simulink model "MPC"  (R2024b)
settings: Solver=ode4  StartTime=0.0  StopTime=tsim  FixedStep=baseRate  RelTol=1e-6  AbsTol=1e-6
values from neighbouring files (symbols this model uses):
  IBLACK = 0.1996    [unpackData.m]
  IRED = 0.1982    [unpackData.m]
  m = m + 5    (= 4)    [unpackData.m]
  M = diag([1/m; 1/m; 1/I])    [unpackData.m]
  mBLACK = 11.3620    (= 11.362)    [unpackData.m]
  mRED = 11.2970    (= 11.297)    [unpackData.m]
  N = 0    [unpackData.m]
  Q = blkdiag(0.0001*eye(2), 0.00001)    [unpackData.m]
  R = diag([6;6;6])    [unpackData.m]
undefined symbols (not defined in the file or in its folder): a1, a2, a3, alpha, alpha_m, alpha_t, alphas, alphas_t, alphat, Am, b, b0, b1, b2, b3, baseRate, Bm, C, c, c1, c1t, c2, c2t, camera_FOV, camera_offset, Cm, d, dataRate, DiscIntNeverNeededParam, Dm, docking_face, docking_offset, drop_states_ARM, drop_states_BLACK, drop_states_BLUE, drop_states_RED, epsilon, epsilont, eta, F_black_X_nominal, F_black_Y_nominal, F_blue_X_nominal, F_blue_Y_nominal, F_max, F_red_X_nominal, F_red_Y_nominal, f_t, F_t, F_thrusters_BLACK, F_thrusters_BLUE, F_thrusters_RED, F_u, f_u, F_v, gamma, Gamma1_el, Gamma1_sh, Gamma1_wr, Gamma2_el, Gamma2_sh ... (+118)
libraries: simulink x33, nvidiaSharedBlocks x13, slpidlib x6, MainLibrary x5, dspsigops x3, dspinverses x3, nvidiaIMUSensorslib x1
(part 6 of 11)

== system MPC/4 - Control/Default PD Control (RED)/Calculate Error ==
  Desired Attitude : Inport
  Measured Attitude : Inport  Port=2
  MATLAB Function : MATLAB Function  TreatAsAtomicUnit=on
  Attitude Error : Outport
  wires:
  MATLAB Function/1(Rz_error) -> Attitude Error/1
  Desired Attitude/1 -> MATLAB Function/1(Rz_path)
  Measured Attitude/1 -> MATLAB Function/2(Rz_measured)

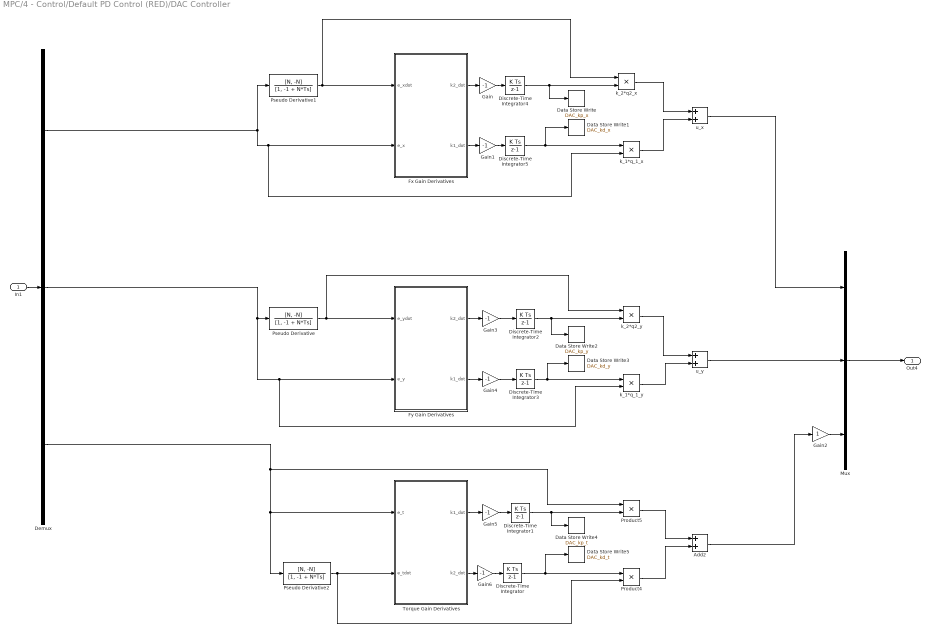
== system MPC/4 - Control/Default PD Control (RED)/DAC Controller ==
  In1 : Inport
  Add2 : Sum
  Data Store Write : DataStoreWrite  DataStoreName=DAC_kp_x  IndexOptions=Index vector (dialog)  Indices=1  OutputSizes=1
  Data Store Write1 : DataStoreWrite  DataStoreName=DAC_kd_x  IndexOptions=Index vector (dialog)  Indices=1  OutputSizes=1
  Data Store Write2 : DataStoreWrite  DataStoreName=DAC_kp_y  IndexOptions=Index vector (dialog)  Indices=1  OutputSizes=1
  Data Store Write3 : DataStoreWrite  DataStoreName=DAC_kd_y  IndexOptions=Index vector (dialog)  Indices=1  OutputSizes=1
  Data Store Write4 : DataStoreWrite  DataStoreName=DAC_kp_t  IndexOptions=Index vector (dialog)  Indices=1  OutputSizes=1
  Data Store Write5 : DataStoreWrite  DataStoreName=DAC_kd_t  IndexOptions=Index vector (dialog)  Indices=1  OutputSizes=1
  Demux : Demux  Outputs=3
  Discrete-Time Integrator : DiscreteIntegrator  InitialCondition=k_2_t_0  SampleTime=-1  ICPrevOutput=DiscIntNeverNeededParam  ICPrevScaledInput=DiscIntNeverNeededParam
  Discrete-Time Integrator1 : DiscreteIntegrator  InitialCondition=k_1_t_0  SampleTime=-1  ICPrevOutput=DiscIntNeverNeededParam  ICPrevScaledInput=DiscIntNeverNeededParam
  Discrete-Time Integrator2 : DiscreteIntegrator  InitialCondition=k_2_0  SampleTime=-1  ICPrevOutput=DiscIntNeverNeededParam  ICPrevScaledInput=DiscIntNeverNeededParam
  Discrete-Time Integrator3 : DiscreteIntegrator  InitialCondition=k_1_0  SampleTime=-1  ICPrevOutput=DiscIntNeverNeededParam  ICPrevScaledInput=DiscIntNeverNeededParam
  Discrete-Time Integrator4 : DiscreteIntegrator  InitialCondition=k_2_0  SampleTime=-1  ICPrevOutput=DiscIntNeverNeededParam  ICPrevScaledInput=DiscIntNeverNeededParam
  Discrete-Time Integrator5 : DiscreteIntegrator  InitialCondition=k_1_0  SampleTime=-1  ICPrevOutput=DiscIntNeverNeededParam  ICPrevScaledInput=DiscIntNeverNeededParam
  Fx Gain Derivatives : MATLAB Function  TreatAsAtomicUnit=on
  Fy Gain Derivatives : MATLAB Function  TreatAsAtomicUnit=on
  Gain{,1,3..6} (6 alike) : Gain  Gain=-1
  Gain2 : Gain
  Mux : Mux  Inputs=3
  Product4 : Product
  Product5 : Product
  Pseudo Derivative : DiscreteTransferFcn  Numerator=[N, -N]  Denominator=[1, -1 + N*Ts]
  Pseudo Derivative1 : DiscreteTransferFcn  Numerator=[N, -N]  Denominator=[1, -1 + N*Ts]
  Pseudo Derivative2 : DiscreteTransferFcn  Numerator=[N, -N]  Denominator=[1, -1 + N*Ts]
  Torque Gain Derivatives : MATLAB Function  TreatAsAtomicUnit=on
  k_1*q_1_x : Product
  k_1*q_1_y : Product
  k_2*q2_x : Product
  k_2*q2_y : Product
  u_x : Sum
  u_y : Sum
  Out4 : Outport
  wires:
  Add2/1 -> Gain2/1
  u_y/1 -> Mux/2
  Pseudo Derivative/1 -> k_2*q2_y/1, Fy Gain Derivatives/1(e_ydot)
  Demux/2 -> Fy Gain Derivatives/2(e_y), k_1*q_1_y/2, Pseudo Derivative/1
  k_2*q2_y/1 -> u_y/1
  Fy Gain Derivatives/2(k1_dot) -> Gain4/1
  k_1*q_1_y/1 -> u_y/2
  Fy Gain Derivatives/1(k2_dot) -> Gain3/1
  Torque Gain Derivatives/1(k1_dot) -> Gain5/1
  Pseudo Derivative2/1 -> Torque Gain Derivatives/2(e_tdot), Product4/2
  Product5/1 -> Add2/1
  Product4/1 -> Add2/2
  Torque Gain Derivatives/2(k2_dot) -> Gain6/1
  Demux/1 -> k_1*q_1_x/2, Fx Gain Derivatives/2(e_x), Pseudo Derivative1/1
  Pseudo Derivative1/1 -> k_2*q2_x/1, Fx Gain Derivatives/1(e_xdot)
  k_1*q_1_x/1 -> u_x/2
  u_x/1 -> Mux/1
  k_2*q2_x/1 -> u_x/1
  Demux/3 -> Torque Gain Derivatives/1(e_t), Pseudo Derivative2/1, Product5/1
  In1/1 -> Demux/1
  Mux/1 -> Out4/1
  Gain2/1 -> Mux/3
  Discrete-Time Integrator2/1 -> Data Store Write2/1, k_2*q2_y/2
  Discrete-Time Integrator5/1 -> Data Store Write1/1, k_1*q_1_x/1
  Discrete-Time Integrator4/1 -> Data Store Write/1, k_2*q2_x/2
  Discrete-Time Integrator1/1 -> Data Store Write4/1, Product5/2
  Fx Gain Derivatives/1(k2_dot) -> Gain/1
  Fx Gain Derivatives/2(k1_dot) -> Gain1/1
  Gain/1 -> Discrete-Time Integrator4/1
  Gain1/1 -> Discrete-Time Integrator5/1
  Gain3/1 -> Discrete-Time Integrator2/1
  Gain4/1 -> Discrete-Time Integrator3/1
  Gain5/1 -> Discrete-Time Integrator1/1
  Gain6/1 -> Discrete-Time Integrator/1
  Discrete-Time Integrator3/1 -> Data Store Write3/1, k_1*q_1_y/1
  Discrete-Time Integrator/1 -> Data Store Write5/1, Product4/1

== system MPC/4 - Control/Default PD Control (RED)/Diff ==
  In1 : Inport
  In2 : Inport  Port=2
  Demux : Demux  Outputs=3
  Demux1 : Demux  Outputs=3
  Hough Control : Subsystem
      settings: PortSchema="{\"entries\":[{\"content\":{\"sides\":[{\"content\":{\"connectorIds\":[\"In1\"]},\"type\":\"ConnectorPlacement.EquallySpacedRectSide\",\"uuid\":\"a8dcddb7-9836-4673-8356-a3c89c9502b3\"},{\"content\":{\"connectorIds\":[\"Out1\"],\"side\":\"RIGHT\"},\"type\":\"ConnectorPlacement.EquallySpacedRectSide\",\"uuid\":\"2c97d3bb-11f9-4ba2-b448-09694ac8e6f8\"},{\"content\":{\"side\":\"TOP\"},\"type\":\"ConnectorPlacement.EquallySpacedRectSide\",\"uuid\":\"bc41882c-3443-497d-b6f8-69c8cbf4c339\"},{\"content\":{\"connectorIds\":[\"In2\"],\"side\":\"BOTTOM\"},\"type\":\"ConnectorPlacement.EquallySpacedRectSide\",\"uuid\":\"14b1077a-07d2-46a7-87f1-61ebe292854a\"}]},\"type\":\"ConnectorPlacement.EquallySpacedConnector\",\"uuid\":\"2f9ed5e7-457a-4e66-9582-5133e2ff8cc8\"}],\"packageUris\":[\"http://schema.mathworks.com/mf0/Connector/R2020b\"],\"version\":\"1.0\"}"
  Mux : Mux  Inputs=3
  Sum : Sum  Inputs=|+-
  Sum1 : Sum  Inputs=|+-
  u : Outport
  wires:
  In1/1 -> Demux/1
  Demux/2 -> Sum/1
  Demux/1 -> Sum1/1
  In2/1 -> Demux1/1
  Demux1/1 -> Sum1/2
  Demux1/2 -> Sum/2
  Demux/3 -> Hough Control/1(Ref)
  Demux1/3 -> Hough Control/2(Act)
  Hough Control/1(Err) -> Mux/3
  Sum/1 -> Mux/2
  Sum1/1 -> Mux/1
  Mux/1 -> u/1

== system MPC/4 - Control/Default PD Control (RED)/H_inf ==
  In1 : Inport
  Demux : Demux  Outputs=3
  Discrete State-Space : DiscreteStateSpace  A=K.A  B=K.B  C=K.C  D=K.D  SampleTime=-1
  Discrete State-Space1 : DiscreteStateSpace  A=K_t.A  B=K_t.B  C=K_t.C  D=K_t.D  SampleTime=-1
  Discrete State-Space2 : DiscreteStateSpace  A=K.A  B=K.B  C=K.C  D=K.D  SampleTime=-1
  Mux : Mux  Inputs=3
  Out1 : Outport
  wires:
  In1/1 -> Demux/1
  Mux/1 -> Out1/1
  Demux/3 -> Discrete State-Space1/1
  Discrete State-Space1/1 -> Mux/3
  Demux/1 -> Discrete State-Space/1
  Discrete State-Space/1 -> Mux/1
  Demux/2 -> Discrete State-Space2/1
  Discrete State-Space2/1 -> Mux/2

== system MPC/4 - Control/Default PD Control (RED)/Homo ==
  In1 : Inport
  Demux : Demux  Outputs=3
  MATLAB Function : MATLAB Function  TreatAsAtomicUnit=on
  MATLAB Function1 : MATLAB Function  TreatAsAtomicUnit=on
  MATLAB Function2 : MATLAB Function  TreatAsAtomicUnit=on
  MATLAB Function3 : MATLAB Function  TreatAsAtomicUnit=on
  MATLAB Function4 : MATLAB Function  TreatAsAtomicUnit=on
  MATLAB Function5 : MATLAB Function  TreatAsAtomicUnit=on
  Mux : Mux  Inputs=3
  Pseudo Derivative : DiscreteTransferFcn  Numerator=[N, -N]  Denominator=[1, -1 + N*Ts]
  Pseudo Derivative1 : DiscreteTransferFcn  Numerator=[N, -N]  Denominator=[1, -1 + N*Ts]
  Pseudo Derivative2 : DiscreteTransferFcn  Numerator=[N, -N]  Denominator=[1, -1 + N*Ts]
  Sum : Sum  Inputs=++|
  Sum1 : Sum  Inputs=++|
  Sum2 : Sum  Inputs=++|
  Out1 : Outport
  wires:
  Demux/1 -> Pseudo Derivative/1, MATLAB Function/1(q1)
  Pseudo Derivative/1 -> MATLAB Function1/1(q2)
  Sum/1 -> Mux/1
  MATLAB Function/1(u) -> Sum/1
  MATLAB Function1/1(u) -> Sum/2
  Pseudo Derivative1/1 -> MATLAB Function3/1(q2)
  Sum1/1 -> Mux/2
  MATLAB Function3/1(u) -> Sum1/2
  Demux/2 -> MATLAB Function2/1(q1), Pseudo Derivative1/1
  MATLAB Function2/1(u) -> Sum1/1
  Demux/3 -> MATLAB Function4/1(q1), Pseudo Derivative2/1
  Pseudo Derivative2/1 -> MATLAB Function5/1(q2)
  MATLAB Function5/1(u) -> Sum2/2
  MATLAB Function4/1(u) -> Sum2/1
  Sum2/1 -> Mux/3
  Mux/1 -> Out1/1
  In1/1 -> Demux/1

== system MPC/4 - Control/Default PD Control (RED)/LQR ==
  In1 : Inport
  Constant : Constant  Value=k
  Demux : Demux  Outputs=3
  MATLAB Function : MATLAB Function  TreatAsAtomicUnit=on
  Pseudo Derivative : DiscreteTransferFcn  Numerator=[N, -N]  Denominator=[1, -1 + N*Ts]
  Pseudo Derivative1 : DiscreteTransferFcn  Numerator=[N, -N]  Denominator=[1, -1 + N*Ts]
  Pseudo Derivative2 : DiscreteTransferFcn  Numerator=[N, -N]  Denominator=[1, -1 + N*Ts]
  Out1 : Outport
  wires:
  Constant/1 -> MATLAB Function/1(k)
  MATLAB Function/1(u) -> Out1/1
  Demux/3 -> Pseudo Derivative2/1, MATLAB Function/6(q1_t)
  Demux/2 -> Pseudo Derivative1/1, MATLAB Function/4(q1_y)
  Demux/1 -> Pseudo Derivative/1, MATLAB Function/2(q1_x)
  Pseudo Derivative2/1 -> MATLAB Function/7(q2_t)
  Pseudo Derivative/1 -> MATLAB Function/3(q2_x)
  Pseudo Derivative1/1 -> MATLAB Function/5(q2_y)
  In1/1 -> Demux/1

== system MPC/4 - Control/Default PD Control (RED)/Min Energy ==
  In1 : Inport
  Clock : Clock
  Clock1 : Clock
  Clock2 : Clock
  Demux : Demux  Outputs=3
  MATLAB Function : MATLAB Function  TreatAsAtomicUnit=on
  MATLAB Function1 : MATLAB Function  TreatAsAtomicUnit=on
  MATLAB Function2 : MATLAB Function  TreatAsAtomicUnit=on
  Mux : Mux  Inputs=3
  Pseudo Derivative : DiscreteTransferFcn  Numerator=[N, -N]  Denominator=[1, -1 + N*Ts]
  Pseudo Derivative1 : DiscreteTransferFcn  Numerator=[N, -N]  Denominator=[1, -1 + N*Ts]
  Pseudo Derivative2 : DiscreteTransferFcn  Numerator=[N, -N]  Denominator=[1, -1 + N*Ts]
  Subsystem : Subsystem
  Subsystem1 : Subsystem
  Subsystem2 : Subsystem
  Sum : Sum  Inputs=|++
  Sum1 : Sum  Inputs=|++
  Sum2 : Sum  Inputs=|++
  Out1 : Outport
  wires:
  Demux/2 -> Subsystem1/2(u), Pseudo Derivative1/1, MATLAB Function/1(q1)
  Pseudo Derivative1/1 -> MATLAB Function/2(q2)
  Clock/1 -> MATLAB Function/3(t)
  MATLAB Function/1(u) -> Sum1/1
  Clock1/1 -> MATLAB Function1/3(t)
  Pseudo Derivative/1 -> MATLAB Function1/2(q2)
  MATLAB Function1/1(u) -> Sum/1
  Demux/1 -> Subsystem/2(u), MATLAB Function1/1(q1), Pseudo Derivative/1
  Clock2/1 -> MATLAB Function2/3(t)
  Pseudo Derivative2/1 -> MATLAB Function2/2(q2)
  MATLAB Function2/1(u) -> Sum2/1
  Demux/3 -> Subsystem2/2(u), Pseudo Derivative2/1, MATLAB Function2/1(q1)
  Mux/1 -> Out1/1
  In1/1 -> Demux/1
  MATLAB Function1/2(dt) -> Subsystem/1(In2)
  Sum/1 -> Mux/1
  Subsystem/1(Out1) -> Sum/2
  MATLAB Function/2(dt) -> Subsystem1/1(dt)
  Sum1/1 -> Mux/2
  Subsystem1/1(Out1) -> Sum1/2
  Sum2/1 -> Mux/3
  Subsystem2/1(Out1) -> Sum2/2
  MATLAB Function2/2(dt) -> Subsystem2/1(dt)

== system MPC/4 - Control/Default PD Control (RED)/Minimum Time Controller ==
  In1 : Inport
  Demux : Demux  Outputs=3
  Gain : Gain  Gain=F_max
  Gain1 : Gain  Gain=F_max
  Gain2 : Gain  Gain=T_max
  MATLAB Function : MATLAB Function  TreatAsAtomicUnit=on
  MATLAB Function1 : MATLAB Function  TreatAsAtomicUnit=on
  MATLAB Function2 : MATLAB Function  TreatAsAtomicUnit=on
  MATLAB Function3 : MATLAB Function  TreatAsAtomicUnit=on
  MATLAB Function4 : MATLAB Function  TreatAsAtomicUnit=on
  MATLAB Function5 : MATLAB Function  TreatAsAtomicUnit=on
  Mux : Mux  Inputs=3
  Pseudo Derivative : DiscreteTransferFcn  Numerator=[N, -N]  Denominator=[1, -1 + N*Ts]
  Pseudo Derivative1 : DiscreteTransferFcn  Numerator=[N, -N]  Denominator=[1, -1 + N*Ts]
  Pseudo Derivative2 : DiscreteTransferFcn  Numerator=[N, -N]  Denominator=[1, -1 + N*Ts]
  Out1 : Outport
  wires:
  Demux/1 -> MATLAB Function/1(q_1), MATLAB Function3/1(q_1), Pseudo Derivative/1
  Demux/3 -> Pseudo Derivative2/1, MATLAB Function2/1(q_1), MATLAB Function5/1(q_1)
  Pseudo Derivative/1 -> MATLAB Function/2(q_2)
  Demux/2 -> Pseudo Derivative1/1, MATLAB Function4/1(q_1), MATLAB Function1/1(q_1)
  Pseudo Derivative1/1 -> MATLAB Function1/2(q_2)
  Pseudo Derivative2/1 -> MATLAB Function2/2(q_2)
  MATLAB Function/1(sign_Argument) -> MATLAB Function3/2(sign_Argument)
  MATLAB Function1/1(sign_Argument) -> MATLAB Function4/2(sign_Argument)
  MATLAB Function2/1(sign_Argument) -> MATLAB Function5/2(sign_Argument)
  MATLAB Function3/1(u_max_product) -> Gain/1
  Gain/1 -> Mux/1
  MATLAB Function4/1(u_max_product) -> Gain1/1
  Gain1/1 -> Mux/2
  MATLAB Function5/1(u_max_product) -> Gain2/1
  Gain2/1 -> Mux/3
  In1/1 -> Demux/1
  Mux/1 -> Out1/1

== system MPC/4 - Control/Default PD Control (RED)/PD ==
  In1 : Inport
  Demux : Demux  Outputs=3
  Mux : Mux  Inputs=3
  PID Controller1 : slpidlib/PID Controller  Controller=PD  Form=Parallel  TimeDomain=Discrete-time  UseExternalTs=off  SampleTime=-1  IntegratorMethod=Forward Euler  FilterMethod=Forward Euler  ControllerParametersSource=internal  P=k_p  I=1  UseKiTs=off  D=k_d  N=N  UseFilter=on  TunerSelectOption=Transfer Function Based (PID Tuner App)  InitialConditionSource=internal  InitialConditionForIntegrator=0  InitialConditionForFilter=0  DifferentiatorICPrevScaledInput=0  ExternalReset=none  TrackingMode=off  Kt=1  LimitOutput=off  SatLimitsSource=internal  UpperSaturationLimit=inf  LowerSaturationLimit=-inf  LinearizeAsGain=on  AntiWindupMode=none  Kb=1  LimitIntegrator=off  UpperIntegratorSaturationLimit=inf  LowerIntegratorSaturationLimit=-inf  POutMin=[]  POutMax=[]  IOutMin=[]  IOutMax=[]  DOutMin=[]  DOutMax=[]  NOutMin=[]  NOutMax=[]  SumOutMin=[]  SumOutMax=[]  SaturationOutMin=[]  SaturationOutMax=[]  PParamMin=[]  PParamMax=[]  IParamMin=[]  IParamMax=[]  DParamMin=[]  DParamMax=[]  NParamMin=[]  NParamMax=[]  KbParamMin=[]  KbParamMax=[]  KtParamMin=[]  KtParamMax=[]  KbOutMin=[]  KbOutMax=[]  KtOutMin=[]  KtOutMax=[]  IntegratorOutMin=[]  IntegratorOutMax=[]  FilterOutMin=[]  FilterOutMax=[]  SumI1OutMin=[]  SumI1OutMax=[]  SumI2OutMin=[]  SumI2OutMax=[]  SumI3OutMin=[]  SumI3OutMax=[]  SumI4OutMin=[]  SumI4OutMax=[]  SumDOutMin=[]  SumDOutMax=[]  DifferentiatorOutMin=[]  DifferentiatorOutMax=[]  FilterDiffOutCoefMin=[]  FilterDiffOutCoefMax=[]  ReciprocalOutMin=[]  ReciprocalOutMax=[]  SumDenOutMin=[]  SumDenOutMax=[]  SumNumOutMin=[]  SumNumOutMax=[]  DivideOutMin=[]  DivideOutMax=[]  UdiffTsProdOutMin=[]  UdiffTsProdOutMax=[]  NTsProdOutMin=[]  NTsProdOutMax=[]  UintegralTsProdOutMin=[]  UintegralTsProdOutMax=[]  UngainTsProdOutMin=[]  UngainTsProdOutMax=[]  ClampingZeroOutDataTypeStr=Inherit: Inherit via back propagation  ClampingZeroOutMin=[]  ClampingZeroOutMax=[]  FilterDenConstantOutDataTypeStr=Inherit: Inherit via back propagation  FilterDenConstantOutMin=[]  FilterDenConstantOutMax=[]  PCopyOutDataTypeStr=Inherit: Inherit via back propagation  PCopyOutMin=[]  PCopyOutMax=[]  NCopyOutDataTypeStr=Inherit: Inherit via back propagation  NCopyOutMin=[]  NCopyOutMax=[]  IntegratorContinuousStateAttributes=''  IntegratorStateMustResolveToSignalObject=off  IntegratorRTWStateStorageClass=Auto  FilterContinuousStateAttributes=''  FilterStateMustResolveToSignalObject=off  FilterRTWStateStorageClass=Auto  ParallelPVariant=InternalParameters  IdealPVariant=Disabled  IVariant=Disabled  DVariant=InternalParameters  IntegratorVariant=Disabled  SatVariant=Disabled  AWVariant=Disabled  PCopyVariant=Disabled  TRVariant=Disabled  FdbkBlocksVariant=Forward  IdealPFdbkVariant=Disabled  SatFdbkVariant=Disabled  DerivativeFilterVariant=ForwardEulerFilter  NVariant=InternalParameters  NCopyVariant=Disabled  FilterICVariant=InternalICsFilter  IntegratorICVariant=Disabled  ExternalResetVariant=Disabled  TRSumVariant=Passthrough  SumFdbkVariant=Disabled  SumVariant=Sum_PD  TsampFilterVariant=InternalTs  TsampNgainVariant=Passthrough  TsampIntegralVariant=Disabled_SignalSpec  ExternalSaturationOutDataTypeStr=Inherit: Same as second input
  PID Controller2 : slpidlib/PID Controller  Controller=PD  Form=Parallel  TimeDomain=Discrete-time  UseExternalTs=off  SampleTime=-1  IntegratorMethod=Forward Euler  FilterMethod=Forward Euler  ControllerParametersSource=internal  P=k_p  I=1  UseKiTs=off  D=k_d  N=N  UseFilter=on  TunerSelectOption=Transfer Function Based (PID Tuner App)  InitialConditionSource=internal  InitialConditionForIntegrator=0  InitialConditionForFilter=0  DifferentiatorICPrevScaledInput=0  ExternalReset=none  TrackingMode=off  Kt=1  LimitOutput=off  SatLimitsSource=internal  UpperSaturationLimit=inf  LowerSaturationLimit=-inf  LinearizeAsGain=on  AntiWindupMode=none  Kb=1  LimitIntegrator=off  UpperIntegratorSaturationLimit=inf  LowerIntegratorSaturationLimit=-inf  POutMin=[]  POutMax=[]  IOutMin=[]  IOutMax=[]  DOutMin=[]  DOutMax=[]  NOutMin=[]  NOutMax=[]  SumOutMin=[]  SumOutMax=[]  SaturationOutMin=[]  SaturationOutMax=[]  PParamMin=[]  PParamMax=[]  IParamMin=[]  IParamMax=[]  DParamMin=[]  DParamMax=[]  NParamMin=[]  NParamMax=[]  KbParamMin=[]  KbParamMax=[]  KtParamMin=[]  KtParamMax=[]  KbOutMin=[]  KbOutMax=[]  KtOutMin=[]  KtOutMax=[]  IntegratorOutMin=[]  IntegratorOutMax=[]  FilterOutMin=[]  FilterOutMax=[]  SumI1OutMin=[]  SumI1OutMax=[]  SumI2OutMin=[]  SumI2OutMax=[]  SumI3OutMin=[]  SumI3OutMax=[]  SumI4OutMin=[]  SumI4OutMax=[]  SumDOutMin=[]  SumDOutMax=[]  DifferentiatorOutMin=[]  DifferentiatorOutMax=[]  FilterDiffOutCoefMin=[]  FilterDiffOutCoefMax=[]  ReciprocalOutMin=[]  ReciprocalOutMax=[]  SumDenOutMin=[]  SumDenOutMax=[]  SumNumOutMin=[]  SumNumOutMax=[]  DivideOutMin=[]  DivideOutMax=[]  UdiffTsProdOutMin=[]  UdiffTsProdOutMax=[]  NTsProdOutMin=[]  NTsProdOutMax=[]  UintegralTsProdOutMin=[]  UintegralTsProdOutMax=[]  UngainTsProdOutMin=[]  UngainTsProdOutMax=[]  ClampingZeroOutDataTypeStr=Inherit: Inherit via back propagation  ClampingZeroOutMin=[]  ClampingZeroOutMax=[]  FilterDenConstantOutDataTypeStr=Inherit: Inherit via back propagation  FilterDenConstantOutMin=[]  FilterDenConstantOutMax=[]  PCopyOutDataTypeStr=Inherit: Inherit via back propagation  PCopyOutMin=[]  PCopyOutMax=[]  NCopyOutDataTypeStr=Inherit: Inherit via back propagation  NCopyOutMin=[]  NCopyOutMax=[]  IntegratorContinuousStateAttributes=''  IntegratorStateMustResolveToSignalObject=off  IntegratorRTWStateStorageClass=Auto  FilterContinuousStateAttributes=''  FilterStateMustResolveToSignalObject=off  FilterRTWStateStorageClass=Auto  ParallelPVariant=InternalParameters  IdealPVariant=Disabled  IVariant=Disabled  DVariant=InternalParameters  IntegratorVariant=Disabled  SatVariant=Disabled  AWVariant=Disabled  PCopyVariant=Disabled  TRVariant=Disabled  FdbkBlocksVariant=Forward  IdealPFdbkVariant=Disabled  SatFdbkVariant=Disabled  DerivativeFilterVariant=ForwardEulerFilter  NVariant=InternalParameters  NCopyVariant=Disabled  FilterICVariant=InternalICsFilter  IntegratorICVariant=Disabled  ExternalResetVariant=Disabled  TRSumVariant=Passthrough  SumFdbkVariant=Disabled  SumVariant=Sum_PD  TsampFilterVariant=InternalTs  TsampNgainVariant=Passthrough  TsampIntegralVariant=Disabled_SignalSpec  ExternalSaturationOutDataTypeStr=Inherit: Same as second input
  PID Controller3 : slpidlib/PID Controller  Controller=PD  Form=Parallel  TimeDomain=Discrete-time  UseExternalTs=off  SampleTime=-1  IntegratorMethod=Forward Euler  FilterMethod=Forward Euler  ControllerParametersSource=internal  P=k_p_t  I=1  UseKiTs=off  D=k_d_t  N=100  UseFilter=on  TunerSelectOption=Transfer Function Based (PID Tuner App)  InitialConditionSource=internal  InitialConditionForIntegrator=0  InitialConditionForFilter=0  DifferentiatorICPrevScaledInput=0  ExternalReset=none  TrackingMode=off  Kt=1  LimitOutput=off  SatLimitsSource=internal  UpperSaturationLimit=inf  LowerSaturationLimit=-inf  LinearizeAsGain=on  AntiWindupMode=none  Kb=1  LimitIntegrator=off  UpperIntegratorSaturationLimit=inf  LowerIntegratorSaturationLimit=-inf  POutMin=[]  POutMax=[]  IOutMin=[]  IOutMax=[]  DOutMin=[]  DOutMax=[]  NOutMin=[]  NOutMax=[]  SumOutMin=[]  SumOutMax=[]  SaturationOutMin=[]  SaturationOutMax=[]  PParamMin=[]  PParamMax=[]  IParamMin=[]  IParamMax=[]  DParamMin=[]  DParamMax=[]  NParamMin=[]  NParamMax=[]  KbParamMin=[]  KbParamMax=[]  KtParamMin=[]  KtParamMax=[]  KbOutMin=[]  KbOutMax=[]  KtOutMin=[]  KtOutMax=[]  IntegratorOutMin=[]  IntegratorOutMax=[]  FilterOutMin=[]  FilterOutMax=[]  SumI1OutMin=[]  SumI1OutMax=[]  SumI2OutMin=[]  SumI2OutMax=[]  SumI3OutMin=[]  SumI3OutMax=[]  SumI4OutMin=[]  SumI4OutMax=[]  SumDOutMin=[]  SumDOutMax=[]  DifferentiatorOutMin=[]  DifferentiatorOutMax=[]  FilterDiffOutCoefMin=[]  FilterDiffOutCoefMax=[]  ReciprocalOutMin=[]  ReciprocalOutMax=[]  SumDenOutMin=[]  SumDenOutMax=[]  SumNumOutMin=[]  SumNumOutMax=[]  DivideOutMin=[]  DivideOutMax=[]  UdiffTsProdOutMin=[]  UdiffTsProdOutMax=[]  NTsProdOutMin=[]  NTsProdOutMax=[]  UintegralTsProdOutMin=[]  UintegralTsProdOutMax=[]  UngainTsProdOutMin=[]  UngainTsProdOutMax=[]  ClampingZeroOutDataTypeStr=Inherit: Inherit via back propagation  ClampingZeroOutMin=[]  ClampingZeroOutMax=[]  FilterDenConstantOutDataTypeStr=Inherit: Inherit via back propagation  FilterDenConstantOutMin=[]  FilterDenConstantOutMax=[]  PCopyOutDataTypeStr=Inherit: Inherit via back propagation  PCopyOutMin=[]  PCopyOutMax=[]  NCopyOutDataTypeStr=Inherit: Inherit via back propagation  NCopyOutMin=[]  NCopyOutMax=[]  IntegratorContinuousStateAttributes=''  IntegratorStateMustResolveToSignalObject=off  IntegratorRTWStateStorageClass=Auto  FilterContinuousStateAttributes=''  FilterStateMustResolveToSignalObject=off  FilterRTWStateStorageClass=Auto  ParallelPVariant=InternalParameters  IdealPVariant=Disabled  IVariant=Disabled  DVariant=InternalParameters  IntegratorVariant=Disabled  SatVariant=Disabled  AWVariant=Disabled  PCopyVariant=Disabled  TRVariant=Disabled  FdbkBlocksVariant=Forward  IdealPFdbkVariant=Disabled  SatFdbkVariant=Disabled  DerivativeFilterVariant=ForwardEulerFilter  NVariant=InternalParameters  NCopyVariant=Disabled  FilterICVariant=InternalICsFilter  IntegratorICVariant=Disabled  ExternalResetVariant=Disabled  TRSumVariant=Passthrough  SumFdbkVariant=Disabled  SumVariant=Sum_PD  TsampFilterVariant=InternalTs  TsampNgainVariant=Passthrough  TsampIntegralVariant=Disabled_SignalSpec  ExternalSaturationOutDataTypeStr=Inherit: Same as second input
  Out1 : Outport
  wires:
  Demux/1 -> PID Controller1/1
  Demux/2 -> PID Controller2/1
  Demux/3 -> PID Controller3/1
  PID Controller3/1 -> Mux/3
  PID Controller1/1 -> Mux/1
  PID Controller2/1 -> Mux/2
  Mux/1 -> Out1/1
  In1/1 -> Demux/1

== system MPC/4 - Control/Default PD Control (RED)/SAC ==
  um : Inport
  States : Inport  Port=2
  Diff : Subsystem
      settings: PortSchema="{\"entries\":[{\"content\":{\"sides\":[{\"content\":{\"connectorIds\":[\"In1\"]},\"type\":\"ConnectorPlacement.EquallySpacedRectSide\",\"uuid\":\"a8dcddb7-9836-4673-8356-a3c89c9502b3\"},{\"content\":{\"connectorIds\":[\"Out1\"],\"side\":\"RIGHT\"},\"type\":\"ConnectorPlacement.EquallySpacedRectSide\",\"uuid\":\"2c97d3bb-11f9-4ba2-b448-09694ac8e6f8\"},{\"content\":{\"side\":\"TOP\"},\"type\":\"ConnectorPlacement.EquallySpacedRectSide\",\"uuid\":\"bc41882c-3443-497d-b6f8-69c8cbf4c339\"},{\"content\":{\"connectorIds\":[\"In2\"],\"side\":\"BOTTOM\"},\"type\":\"ConnectorPlacement.EquallySpacedRectSide\",\"uuid\":\"b35c17fe-b4c8-48b8-8d35-23ad00086ed4\"}]},\"type\":\"ConnectorPlacement.EquallySpacedConnector\",\"uuid\":\"2f9ed5e7-457a-4e66-9582-5133e2ff8cc8\"}],\"packageUris\":[\"http://schema.mathworks.com/mf0/Connector/R2020b\"],\"version\":\"1.0\"}"
  Ideal Plant Model1 : Subsystem  Commented=on
  Ideal Plant Model2 : Subsystem  Commented=on
  Ideal Plant Model3 : Subsystem
  Plant Output : Subsystem
  SAC_CTL : Subsystem
  u : Outport
  wires:
  SAC_CTL/1(u) -> u/1
  States/1 -> Plant Output/1(States)
  um/1 -> Ideal Plant Model3/1(um), SAC_CTL/1(um)
  Ideal Plant Model3/2(ym) -> Diff/1(In1)
  Plant Output/1(u) -> Diff/2(In2)
  Diff/1(u) -> SAC_CTL/3(ey)
  Ideal Plant Model3/1(xm) -> SAC_CTL/2(xm)

== system MPC/4 - Control/Default PD Control (RED)/SMC ==
  In1 : Inport
  Demux : Demux  Outputs=3
  MATLAB Function : MATLAB Function  TreatAsAtomicUnit=on
  MATLAB Function1 : MATLAB Function  TreatAsAtomicUnit=on
  MATLAB Function2 : MATLAB Function  TreatAsAtomicUnit=on
  Mux : Mux  Inputs=3
  Pseudo Derivative : DiscreteTransferFcn  Numerator=[N, -N]  Denominator=[1, -1 + N*Ts]
  Pseudo Derivative1 : DiscreteTransferFcn  Numerator=[N, -N]  Denominator=[1, -1 + N*Ts]
  Pseudo Derivative2 : DiscreteTransferFcn  Numerator=[N, -N]  Denominator=[1, -1 + N*Ts]
  Out1 : Outport
  wires:
  Demux/3 -> MATLAB Function2/1(e), Pseudo Derivative2/1
  Demux/2 -> MATLAB Function1/1(e), Pseudo Derivative1/1
  Demux/1 -> MATLAB Function/1(e), Pseudo Derivative/1
  Pseudo Derivative2/1 -> MATLAB Function2/2(de)
  MATLAB Function2/1(u) -> Mux/3
  Pseudo Derivative1/1 -> MATLAB Function1/2(de)
  MATLAB Function1/1(u) -> Mux/2
  MATLAB Function/1(u) -> Mux/1
  Pseudo Derivative/1 -> MATLAB Function/2(de)
  Mux/1 -> Out1/1
  In1/1 -> Demux/1

== system MPC/4 - Control/Default PD Control (RED)/Sat ==
  In1 : Inport
  Demux : Demux  Outputs=3
  MATLAB Function : MATLAB Function  TreatAsAtomicUnit=on
  MATLAB Function1 : MATLAB Function  TreatAsAtomicUnit=on
  MATLAB Function2 : MATLAB Function  TreatAsAtomicUnit=on
  MATLAB Function3 : MATLAB Function  TreatAsAtomicUnit=on
  MATLAB Function4 : MATLAB Function  TreatAsAtomicUnit=on
  MATLAB Function5 : MATLAB Function  TreatAsAtomicUnit=on
  Mux : Mux  Inputs=3
  Pseudo Derivative : DiscreteTransferFcn  Numerator=[N, -N]  Denominator=[1, -1 + N*Ts]
  Pseudo Derivative1 : DiscreteTransferFcn  Numerator=[N, -N]  Denominator=[1, -1 + N*Ts]
  Pseudo Derivative2 : DiscreteTransferFcn  Numerator=[N, -N]  Denominator=[1, -1 + N*Ts]
  Out1 : Outport
  wires:
  Demux/1 -> Pseudo Derivative/1, MATLAB Function/2(q1)
  Pseudo Derivative1/1 -> MATLAB Function4/1(q2), MATLAB Function1/1(q2)
  Demux/3 -> MATLAB Function2/2(q1), Pseudo Derivative2/1
  Pseudo Derivative2/1 -> MATLAB Function5/1(q2), MATLAB Function2/1(q2)
  Pseudo Derivative/1 -> MATLAB Function3/1(q2), MATLAB Function/1(q2)
  MATLAB Function/1(saturation) -> MATLAB Function3/2(u)
  MATLAB Function2/1(saturation) -> MATLAB Function5/2(u)
  MATLAB Function1/1(saturation) -> MATLAB Function4/2(u)
  MATLAB Function3/1(saturation) -> Mux/1
  MATLAB Function4/1(saturation) -> Mux/2
  MATLAB Function5/1(saturation) -> Mux/3
  Mux/1 -> Out1/1
  In1/1 -> Demux/1
  Demux/2 -> Pseudo Derivative1/1, MATLAB Function1/2(q1)

== system MPC/4 - Control/Default PD Control (RED)/USC ==
  In1 : Inport
  Demux : Demux  Outputs=3
  Discrete-Time Integrator : DiscreteIntegrator  InitialCondition=k_0  SampleTime=-1  ICPrevOutput=DiscIntNeverNeededParam  ICPrevScaledInput=DiscIntNeverNeededParam
  Discrete-Time Integrator1 : DiscreteIntegrator  InitialCondition=k_0  SampleTime=-1  ICPrevOutput=DiscIntNeverNeededParam  ICPrevScaledInput=DiscIntNeverNeededParam
  Discrete-Time Integrator2 : DiscreteIntegrator  InitialCondition=kt_0  SampleTime=-1  ICPrevOutput=DiscIntNeverNeededParam  ICPrevScaledInput=DiscIntNeverNeededParam
  Gain : Gain  Gain=-1
  MATLAB Function : MATLAB Function  TreatAsAtomicUnit=on
  MATLAB Function1 : MATLAB Function  TreatAsAtomicUnit=on
  MATLAB Function2 : MATLAB Function  TreatAsAtomicUnit=on
  MATLAB Function3 : MATLAB Function  TreatAsAtomicUnit=on
  MATLAB Function4 : MATLAB Function  TreatAsAtomicUnit=on
  MATLAB Function5 : MATLAB Function  TreatAsAtomicUnit=on
  Mux : Mux  Inputs=3
  Pseudo Derivative : DiscreteTransferFcn  Numerator=[N, -N]  Denominator=[1, -1 + N*Ts]
  Pseudo Derivative1 : DiscreteTransferFcn  Numerator=[N, -N]  Denominator=[1, -1 + N*Ts]
  Pseudo Derivative2 : DiscreteTransferFcn  Numerator=[N, -N]  Denominator=[1, -1 + N*Ts]
  RED_Fx : DataStoreWrite  DataStoreName=USC_k_x  IndexOptions=Index vector (dialog)  Indices=1  OutputSizes=1
  RED_Fy : DataStoreWrite  DataStoreName=USC_k_y  IndexOptions=Index vector (dialog)  Indices=1  OutputSizes=1
  RED_Tz : DataStoreWrite  DataStoreName=USC_k_t  IndexOptions=Index vector (dialog)  Indices=1  OutputSizes=1
  Out1 : Outport
  wires:
  In1/1 -> Demux/1
  MATLAB Function/1(k_dot) -> Discrete-Time Integrator/1
  Discrete-Time Integrator/1 -> RED_Fx/1, MATLAB Function1/1(k)
  MATLAB Function1/1(u) -> Mux/1
  Pseudo Derivative/1 -> MATLAB Function1/2(q2), MATLAB Function/2(q2)
  Discrete-Time Integrator1/1 -> MATLAB Function3/1(k), RED_Fy/1
  Demux/2 -> Pseudo Derivative1/1, MATLAB Function3/3(q1), MATLAB Function2/1(q1)
  MATLAB Function2/1(k_dot) -> Discrete-Time Integrator1/1
  Pseudo Derivative1/1 -> MATLAB Function3/2(q2), MATLAB Function2/2(q2)
  Discrete-Time Integrator2/1 -> RED_Tz/1, MATLAB Function5/1(k)
  Pseudo Derivative2/1 -> MATLAB Function5/2(q2), MATLAB Function4/2(q2)
  MATLAB Function4/1(k_dot) -> Discrete-Time Integrator2/1
  Demux/3 -> Pseudo Derivative2/1, MATLAB Function5/3(q1), MATLAB Function4/1(q1)
  Mux/1 -> Gain/1
  Gain/1 -> Out1/1
  MATLAB Function3/1(u) -> Mux/2
  MATLAB Function5/1(u) -> Mux/3
  Demux/1 -> MATLAB Function/1(q1), MATLAB Function1/3(q1), Pseudo Derivative/1

== system MPC/Model Predictive Control/Model Predictive Control/Retrieve BLACK State ==
  Data Store Read : DataStoreRead  DataStoreName=BLACK_Measured_States_RAW  IndexOptions=Index vector (dialog)  Indices=1  OutputSizes=1
  Demux : Demux  Outputs=[2,1,3,3]
  Mux : Mux  Inputs=[2,1,3]
  Terminator : Terminator
  Unwrap1 : dspsigops/Unwrap  tol=pi  InputProcessing=Columns as channels (frame based)  running=off
  x_BLACK : Outport
  wires:
  Data Store Read/1 -> Demux/1
  Demux/2 -> Unwrap1/1
  Demux/1 -> Mux/1
  Unwrap1/1 -> Mux/2
  Mux/1 -> x_BLACK/1
  Demux/3 -> Mux/3
  Demux/4 -> Terminator/1

== system MPC/Model Predictive Control/Model Predictive Control/Retrieve BLUE State ==
  Data Store Read2 : DataStoreRead  DataStoreName=BLUE_Measured_States  IndexOptions=Index vector (dialog)  Indices=1  OutputSizes=1
  Demux : Demux  Outputs=[2,1,3,3]
  Mux : Mux  Inputs=[2,1,3]
  Terminator : Terminator
  Unwrap1 : dspsigops/Unwrap  tol=pi  InputProcessing=Columns as channels (frame based)  running=off
  x_BLUE : Outport
  wires:
  Data Store Read2/1 -> Demux/1
  Demux/2 -> Unwrap1/1
  Demux/1 -> Mux/1
  Unwrap1/1 -> Mux/2
  Mux/1 -> x_BLUE/1
  Demux/3 -> Mux/3
  Demux/4 -> Terminator/1

== system MPC/Model Predictive Control/Model Predictive Control/Retrieve RED State ==
  Data Store Read : DataStoreRead  DataStoreName=RED_Measured_States_RAW  IndexOptions=Index vector (dialog)  Indices=1  OutputSizes=1
  Demux : Demux  Outputs=[2,1,3,3]
  Mux : Mux  Inputs=[2,1,3]
  Scope : Scope  NumInputPorts=2
  Terminator : Terminator
  Unwrap1 : dspsigops/Unwrap  tol=pi  InputProcessing=Columns as channels (frame based)  running=off
  x_RED : Outport
  wires:
  Unwrap1/1 -> Scope/2, Mux/2  "g"
  Demux/3 -> Mux/3
  Demux/2 -> Scope/1, Unwrap1/1  "f"
  Demux/4 -> Terminator/1
  Mux/1 -> x_RED/1
  Demux/1 -> Mux/1
  Data Store Read/1 -> Demux/1

== system MPC/PhaseSpace Camera Code/Use Hardware to Obtain States/Receive and Process Phasespace Data ==
  "Adjust Time " : Subsystem
  Check for Sychronization : Subsystem
  Clock : Clock
  Demux2 : Demux  Outputs=[1,18]
  Mux : Mux  Inputs=2
  Receive PhaseSpace Data : nvidiaSharedBlocks/UDP Receive  localURL='0.0.0.0'  localPort=31534  remoteURL='0.0.0.0'  remotePort=-1  recvBufferSize=8192  signalDatatype=double  dims=19  isVarSize=off  showBlockingTime=off  blockingTime=0  sampletime=-1  blockPlatform=NVIDIA
  Reshape : Reshape  OutputDimensionality=Customize  OutputDimensions=[19,1]
  Terminator : Terminator
  PhaseSpace Data : Outport
  PhaseSpace Clock : Outport  Port=2
  wires:
  Check for Sychronization/1(StartClock) -> "Adjust Time "/1(ClockStart)
  Reshape/1 -> Demux2/1
  "Adjust Time "/1(ClockAdjusted) -> Mux/1
  Demux2/2 -> Mux/2
  Mux/1 -> PhaseSpace Data/1
  Receive PhaseSpace Data/2 -> Terminator/1
  Receive PhaseSpace Data/1 -> Reshape/1
  Clock/1 -> "Adjust Time "/2(ClockRaw)
  Demux2/1 -> PhaseSpace Clock/1

== system MPC/PhaseSpace Camera Code/Use Hardware to Obtain States/Store BLACK Data ==
  note: Store BLACK Positions and Velocities
  BLACK Data : Inport
  BLACK Velocities : Inport  Port=2
  PS Clock : Inport  Port=3
  Calculate True Time Step : Subsystem
      settings: PortSchema="{\"entries\":[{\"content\":{\"sides\":[{\"content\":{\"connectorIds\":[\"In1\"]},\"type\":\"ConnectorPlacement.EquallySpacedRectSide\",\"uuid\":\"62932c5c-f2a7-44c8-96b4-4a75bab3a126\"},{\"content\":{\"connectorIds\":[\"Out1\"],\"side\":\"RIGHT\"},\"type\":\"ConnectorPlacement.EquallySpacedRectSide\",\"uuid\":\"82b3b717-2171-4047-b0df-3cd41cf9dfc7\"},{\"content\":{\"side\":\"TOP\"},\"type\":\"ConnectorPlacement.EquallySpacedRectSide\",\"uuid\":\"a142272a-a0ff-4882-8a2d-4633b3c7e02f\"},{\"content\":{\"connectorIds\":[\"In2\"],\"side\":\"BOTTOM\"},\"type\":\"ConnectorPlacement.EquallySpacedRectSide\",\"uuid\":\"b1e1ff4c-66d6-488f-92fb-77f76780833b\"}]},\"type\":\"ConnectorPlacement.EquallySpacedConnector\",\"uuid\":\"98c51868-8a10-4b52-aae4-56f6042c65c4\"}],\"packageUris\":[\"http://schema.mathworks.com/mf0/Connector/R2020b\"],\"version\":\"1.0\"}"
  Convert BLACKVX from [mm] to [m] : Gain  Gain=1/1000
  Convert BLACKVY from [mm] to [m] : Gain  Gain=1/1000
  Convert BLAX from [mm] to [m] : Gain  Gain=1/1000
  Convert BLAY from [mm] to [m] : Gain  Gain=1/1000
  Data Store Write : DataStoreWrite  DataStoreName=BLACK_Measured_States_RAW  IndexOptions=Index vector (dialog)  Indices=1  OutputSizes=1
  Demux : Demux  Outputs=3
  Demux2 : Demux  Outputs=3
  Demux3 : Demux  Outputs=3
  Mux{1..4} (4 alike) : Mux  Inputs=3
  Reshape : Reshape  OutputDimensionality=Column vector (2-D)
  Subsystem1 : Subsystem
  Subsystem2 : Subsystem
  Wrap : Subsystem
  wires:
  Demux3/1 -> Convert BLAX from [mm] to [m]/1
  Demux3/2 -> Convert BLAY from [mm] to [m]/1
  BLACK Data/1 -> Demux3/1
  Demux/3 -> Wrap/1(Unwrapped Angle)
  Reshape/1 -> Subsystem1/2(y)
  Demux/1 -> Mux1/1
  Convert BLAY from [mm] to [m]/1 -> Mux3/2
  Calculate True Time Step/1(dt_out) -> Subsystem2/1(dt), Subsystem1/1(dt)
  Mux3/1 -> Subsystem2/2(y), Demux/1, Calculate True Time Step/2(Data)
  Wrap/1(Wrapped Angle) -> Mux1/3
  Convert BLAX from [mm] to [m]/1 -> Mux3/1
  Mux2/1 -> Data Store Write/1
  Demux/2 -> Mux1/2
  Subsystem2/1(dy/dt) -> Reshape/1
  PS Clock/1 -> Calculate True Time Step/1(Time)
  Demux3/3 -> Mux3/3
  Mux1/1 -> Mux2/1
  Subsystem1/1(dy/dt) -> Mux2/3
  BLACK Velocities/1 -> Demux2/1
  Demux2/3 -> Mux4/3
  Convert BLACKVX from [mm] to [m]/1 -> Mux4/1
  Convert BLACKVY from [mm] to [m]/1 -> Mux4/2
  Mux4/1 -> Mux2/2
  Demux2/2 -> Convert BLACKVY from [mm] to [m]/1
  Demux2/1 -> Convert BLACKVX from [mm] to [m]/1

== system MPC/PhaseSpace Camera Code/Use Hardware to Obtain States/Store BLUE Data ==
  note: Store BLUE Positions and Velocities
  BLUE Data : Inport
  BLUE Velocities : Inport  Port=2
  PS Clock : Inport  Port=3
  Calculate True Time Step : Subsystem
      settings: PortSchema="{\"entries\":[{\"content\":{\"sides\":[{\"content\":{\"connectorIds\":[\"In1\"]},\"type\":\"ConnectorPlacement.EquallySpacedRectSide\",\"uuid\":\"62932c5c-f2a7-44c8-96b4-4a75bab3a126\"},{\"content\":{\"connectorIds\":[\"Out1\"],\"side\":\"RIGHT\"},\"type\":\"ConnectorPlacement.EquallySpacedRectSide\",\"uuid\":\"82b3b717-2171-4047-b0df-3cd41cf9dfc7\"},{\"content\":{\"side\":\"TOP\"},\"type\":\"ConnectorPlacement.EquallySpacedRectSide\",\"uuid\":\"a142272a-a0ff-4882-8a2d-4633b3c7e02f\"},{\"content\":{\"connectorIds\":[\"In2\"],\"side\":\"BOTTOM\"},\"type\":\"ConnectorPlacement.EquallySpacedRectSide\",\"uuid\":\"b1e1ff4c-66d6-488f-92fb-77f76780833b\"}]},\"type\":\"ConnectorPlacement.EquallySpacedConnector\",\"uuid\":\"98c51868-8a10-4b52-aae4-56f6042c65c4\"}],\"packageUris\":[\"http://schema.mathworks.com/mf0/Connector/R2020b\"],\"version\":\"1.0\"}"
  Convert BLUEVX from [mm] to [m] : Gain  Gain=1/1000
  Convert BLUEVY from [mm] to [m] : Gain  Gain=1/1000
  Convert BLUX from [mm] to [m] : Gain  Gain=1/1000
  Convert BLUY from [mm] to [m] : Gain  Gain=1/1000
  Data Store Write : DataStoreWrite  DataStoreName=BLUE_Measured_States_RAW  IndexOptions=Index vector (dialog)  Indices=1  OutputSizes=1
  Demux : Demux  Outputs=3
  Demux2 : Demux  Outputs=3
  Demux5 : Demux  Outputs=3
  Mux{1..4} (4 alike) : Mux  Inputs=3
  Reshape : Reshape  OutputDimensionality=Column vector (2-D)
  Subsystem1 : Subsystem
  Subsystem2 : Subsystem
  Wrap : Subsystem
  wires:
  Demux5/2 -> Convert BLUY from [mm] to [m]/1
  Demux5/1 -> Convert BLUX from [mm] to [m]/1
  BLUE Data/1 -> Demux5/1
  Calculate True Time Step/1(dt_out) -> Subsystem2/1(dt), Subsystem1/1(dt)
  Demux/2 -> Mux1/2
  Demux/1 -> Mux1/1
  Subsystem2/1(dy/dt) -> Reshape/1
  Mux3/1 -> Subsystem2/2(y), Demux/1, Calculate True Time Step/2(Data)
  Demux/3 -> Wrap/1(Unwrapped Angle)
  Reshape/1 -> Subsystem1/2(y)
  Wrap/1(Wrapped Angle) -> Mux1/3
  Mux2/1 -> Data Store Write/1
  Convert BLUY from [mm] to [m]/1 -> Mux3/2
  Convert BLUX from [mm] to [m]/1 -> Mux3/1
  Demux5/3 -> Mux3/3
  PS Clock/1 -> Calculate True Time Step/1(Time)
  Mux1/1 -> Mux2/1
  Subsystem1/1(dy/dt) -> Mux2/3
  Demux2/1 -> Convert BLUEVX from [mm] to [m]/1
  Convert BLUEVY from [mm] to [m]/1 -> Mux4/2
  BLUE Velocities/1 -> Demux2/1
  Demux2/2 -> Convert BLUEVY from [mm] to [m]/1
  Mux4/1 -> Mux2/2
  Demux2/3 -> Mux4/3
  Convert BLUEVX from [mm] to [m]/1 -> Mux4/1

== system MPC/PhaseSpace Camera Code/Use Hardware to Obtain States/Store RED Data ==
  note: Store RED Position and Velocity Data
  RED Data : Inport
  RED Velocities : Inport  Port=2
  PS Clock : Inport  Port=3
  Calculate True Time Step : Subsystem
      settings: PortSchema="{\"entries\":[{\"content\":{\"sides\":[{\"content\":{\"connectorIds\":[\"In1\"]},\"type\":\"ConnectorPlacement.EquallySpacedRectSide\",\"uuid\":\"62932c5c-f2a7-44c8-96b4-4a75bab3a126\"},{\"content\":{\"connectorIds\":[\"Out1\"],\"side\":\"RIGHT\"},\"type\":\"ConnectorPlacement.EquallySpacedRectSide\",\"uuid\":\"82b3b717-2171-4047-b0df-3cd41cf9dfc7\"},{\"content\":{\"side\":\"TOP\"},\"type\":\"ConnectorPlacement.EquallySpacedRectSide\",\"uuid\":\"a142272a-a0ff-4882-8a2d-4633b3c7e02f\"},{\"content\":{\"connectorIds\":[\"In2\"],\"side\":\"BOTTOM\"},\"type\":\"ConnectorPlacement.EquallySpacedRectSide\",\"uuid\":\"b1e1ff4c-66d6-488f-92fb-77f76780833b\"}]},\"type\":\"ConnectorPlacement.EquallySpacedConnector\",\"uuid\":\"98c51868-8a10-4b52-aae4-56f6042c65c4\"}],\"packageUris\":[\"http://schema.mathworks.com/mf0/Connector/R2020b\"],\"version\":\"1.0\"}"
  Convert REDVX from [mm] to [m] : Gain  Gain=1/1000
  Convert REDVY from [mm] to [m] : Gain  Gain=1/1000
  Convert REDX from [mm] to [m] : Gain  Gain=1/1000
  Convert REDY from [mm] to [m] : Gain  Gain=1/1000
  Data Store Write : DataStoreWrite  DataStoreName=RED_Measured_States_RAW  IndexOptions=Index vector (dialog)  Indices=1  OutputSizes=1
  Demux : Demux  Outputs=3
  Demux1 : Demux
  Demux2 : Demux  Outputs=3
  Mux{1..4} (4 alike) : Mux  Inputs=3
  Reshape : Reshape  OutputDimensionality=Column vector (2-D)
  Subsystem1 : Subsystem
  Subsystem2 : Subsystem
  Universal_Time : DataStoreWrite  DataStoreName=Univ_Time  IndexOptions=Index vector (dialog)  Indices=1  OutputSizes=1
  Wrap : Subsystem
  wires:
  Demux1/2 -> Convert REDX from [mm] to [m]/1
  Demux1/3 -> Convert REDY from [mm] to [m]/1
  RED Data/1 -> Demux1/1
  Demux1/4 -> Mux3/3
  Demux1/1 -> Universal_Time/1
  Mux2/1 -> Data Store Write/1
  Reshape/1 -> Subsystem1/2(y)
  Wrap/1(Wrapped Angle) -> Mux1/3
  Demux/3 -> Wrap/1(Unwrapped Angle)
  Demux/1 -> Mux1/1
  Subsystem2/1(dy/dt) -> Reshape/1
  Mux3/1 -> Subsystem2/2(y), Demux/1, Calculate True Time Step/2(Data)
  Demux/2 -> Mux1/2
  Convert REDX from [mm] to [m]/1 -> Mux3/1
  Convert REDY from [mm] to [m]/1 -> Mux3/2
  Calculate True Time Step/1(dt_out) -> Subsystem2/1(dt), Subsystem1/1(dt)
  Mux1/1 -> Mux2/1
  Subsystem1/1(dy/dt) -> Mux2/3
  Convert REDVX from [mm] to [m]/1 -> Mux4/1
  Convert REDVY from [mm] to [m]/1 -> Mux4/2
  Demux2/1 -> Convert REDVX from [mm] to [m]/1
  Demux2/2 -> Convert REDVY from [mm] to [m]/1
  Demux2/3 -> Mux4/3
  RED Velocities/1 -> Demux2/1
  Mux4/1 -> Mux2/2
  PS Clock/1 -> Calculate True Time Step/1(Time)

== system MPC/PhaseSpace Filter Code/Subsystem1/Subsystem ==
  u : Inport
  Delay2 : Delay  DelayLength=1
  MATLAB Function1 : MATLAB Function  TreatAsAtomicUnit=on
  y : Outport
  wires:
  u/1 -> Delay2/1, MATLAB Function1/1(u)
  MATLAB Function1/1(y) -> y/1
  Delay2/1 -> MATLAB Function1/2(uprev)

== system MPC/PhaseSpace Filter Code/Subsystem2/Subsystem ==
  u : Inport
  Delay2 : Delay  DelayLength=1
  MATLAB Function1 : MATLAB Function  TreatAsAtomicUnit=on
  y : Outport
  wires:
  Delay2/1 -> MATLAB Function1/2(uprev)
  MATLAB Function1/1(y) -> y/1
  u/1 -> MATLAB Function1/1(u), Delay2/1

== system MPC/PhaseSpace Filter Code/Subsystem3/Subsystem ==
  u : Inport
  Delay2 : Delay  DelayLength=1
  MATLAB Function1 : MATLAB Function  TreatAsAtomicUnit=on
  y : Outport
  wires:
  u/1 -> Delay2/1, MATLAB Function1/1(u)
  MATLAB Function1/1(y) -> y/1
  Delay2/1 -> MATLAB Function1/2(uprev)

== system MPC/Receive Data /Subsystem/Pose1 ==
  yaw : Inport
  x : Inport  Port=2
  MATLAB Function : MATLAB Function  TreatAsAtomicUnit=on
  dq : Outport
  q : Outport  Port=2
  R : Outport  Port=3
  wires:
  x/1 -> MATLAB Function/1(x)
  MATLAB Function/3(R) -> R/1
  MATLAB Function/2(q) -> q/1
  MATLAB Function/1(dq) -> dq/1
  yaw/1 -> MATLAB Function/2(yaw)

== system MPC/Receive Data /Subsystem/Pose2 ==
  yaw : Inport
  x : Inport  Port=2
  MATLAB Function : MATLAB Function  TreatAsAtomicUnit=on
  dq : Outport
  q : Outport  Port=2
  R : Outport  Port=3
  wires:
  yaw/1 -> MATLAB Function/2(yaw)
  MATLAB Function/1(dq) -> dq/1
  MATLAB Function/2(q) -> q/1
  MATLAB Function/3(R) -> R/1
  x/1 -> MATLAB Function/1(x)

== system MPC/Simulate Plant Dynamics/BLACK Dynamics/Calculated & Store Measured States ==
  y : Inport
  dt : Inport  Port=2
  Data Store Write : DataStoreWrite  DataStoreName=BLACK_Measured_States_RAW  IndexOptions=Index vector (dialog)  Indices=1  OutputSizes=1
  Data Store Write7 : DataStoreWrite  Commented=on  DataStoreName=BLACK_Measured_States  IndexOptions=Index vector (dialog)  Indices=1  OutputSizes=1
  Demux : Demux  Outputs=3
  Mux1 : Mux  Inputs=3
  Mux2 : Mux  Inputs=3
  Reshape : Reshape  OutputDimensionality=Column vector (2-D)
  Subsystem1 : Subsystem
  Subsystem2 : Subsystem
  Wrap : Subsystem
  wires:
  Demux/1 -> Mux1/1
  Wrap/1(Wrapped Angle) -> Mux1/3
  Demux/3 -> Wrap/1(Unwrapped Angle)
  Demux/2 -> Mux1/2
  Mux2/1 -> Data Store Write7/1, Data Store Write/1
  Reshape/1 -> Subsystem1/2(y)
  Subsystem2/1(dy/dt) -> Mux2/2, Reshape/1
  y/1 -> Subsystem2/2(y), Demux/1
  Mux1/1 -> Mux2/1
  Subsystem1/1(dy/dt) -> Mux2/3
  dt/1 -> Subsystem1/1(dt), Subsystem2/1(dt)

== system MPC/Simulate Plant Dynamics/BLACK Dynamics/Calculated & Store True States ==
  y : Inport
  Demux : Demux  Outputs=3
  Discrete Derivative : simulink/Discrete/Discrete Derivative  gainval=1.0  ICPrevScaledInput=0.0  OutMin=[]  OutMax=[]  OutDataType=fixdt(1, 16)  OutScaling=2^-10  DoSatur=off
  Discrete Derivative1 : simulink/Discrete/Discrete Derivative  gainval=1.0  ICPrevScaledInput=0.0  OutMin=[]  OutMax=[]  OutDataType=fixdt(1, 16)  OutScaling=2^-10  DoSatur=off
  Mux1 : Mux  Inputs=3
  Mux2 : Mux  Inputs=3
  True States for BLACK : DataStoreWrite  DataStoreName=BLACK_True_States  IndexOptions=Index vector (dialog)  Indices=1  OutputSizes=1
  Wrap : Subsystem
  wires:
  Demux/1 -> Mux1/1
  Wrap/1(Wrapped Angle) -> Mux1/3
  Demux/3 -> Wrap/1(Unwrapped Angle)
  Demux/2 -> Mux1/2
  Mux2/1 -> True States for BLACK/1
  y/1 -> Discrete Derivative/1, Demux/1
  Discrete Derivative/1 -> Mux2/2, Discrete Derivative1/1
  Mux1/1 -> Mux2/1
  Discrete Derivative1/1 -> Mux2/3

== system MPC/Simulate Plant Dynamics/BLACK Dynamics/Data @ Measurement Rate ==
  Data Input : Inport
  Calculate True Time Step : Subsystem
  Constant1 : Constant  Value=dataRate
  Constant2 : Constant  Value=0
  Data Store Read : DataStoreRead  DataStoreName=Univ_Time  IndexOptions=Index vector (dialog)  Indices=1  OutputSizes=1
  Delay : Delay  DelayLength=1
  Enabled Subsystem : Subsystem  TreatAsAtomicUnit=on
  Enabled Subsystem1 : Subsystem  TreatAsAtomicUnit=on
  Relational Operator1 : RelationalOperator  OutDataTypeStr=boolean  RndMeth=Simplest  InputSameDT=off
  Relational Operator2 : RelationalOperator  Operator===  OutDataTypeStr=boolean  RndMeth=Simplest  InputSameDT=off
  Subtract : Sum  Inputs=+-
  Data Held : Outport
  Time Step : Outport  Port=2
  wires:
  Data Input/1 -> Enabled Subsystem1/1(ThrustPer_Final)
  Subtract/1 -> Relational Operator2/1, Delay/1
  Relational Operator2/1 -> Enabled Subsystem1/Enable
  Relational Operator1/1 -> Enabled Subsystem/Enable
  Constant1/1 -> Calculate True Time Step/3(Rate), Relational Operator1/2
  Constant2/1 -> Relational Operator2/2
  Enabled Subsystem/1(Out1) -> Calculate True Time Step/2(Time), Subtract/2
  Delay/1 -> Relational Operator1/1
  Data Store Read/1 -> Enabled Subsystem/1(In1), Subtract/1
  Enabled Subsystem1/1(Out1) -> Calculate True Time Step/1(Data), Data Held/1
  Calculate True Time Step/1(dt_out) -> Time Step/1

== system MPC/Simulate Plant Dynamics/BLACK Dynamics/Dynamics Model for BLACK ==
  control_inputs : Inport
  Acceleration to Velocity : DiscreteIntegrator  IntegratorMethod=Integration: Backward Euler  SampleTime=-1  ICPrevOutput=DiscIntNeverNeededParam  ICPrevScaledInput=DiscIntNeverNeededParam
  Add Noise : RandomNumber  Variance=1e-9  SampleTime=baseRate
  MATLAB Function : MATLAB Function  TreatAsAtomicUnit=on
  Sum : Sum  Inputs=++|
  Velocity to Position : DiscreteIntegrator  IntegratorMethod=Integration: Backward Euler  InitialCondition=drop_states_BLACK  SampleTime=-1  ICPrevOutput=DiscIntNeverNeededParam  ICPrevScaledInput=DiscIntNeverNeededParam
  states : Outport  VectorParamsAs1DForOutWhenUnconnected=off
  wires:
  control_inputs/1 -> MATLAB Function/1(control_inputs)
  Acceleration to Velocity/1 -> Velocity to Position/1
  Velocity to Position/1 -> states/1
  Add Noise/1 -> Sum/1
  MATLAB Function/1(x_ddot) -> Sum/2
  Sum/1 -> Acceleration to Velocity/1

== system MPC/Simulate Plant Dynamics/BLUE Dynamics/BLUE  Dynamics Model ==
  control_inputs : Inport
  Acceleration to Velocity : DiscreteIntegrator  IntegratorMethod=Integration: Backward Euler  SampleTime=-1  ICPrevOutput=DiscIntNeverNeededParam  ICPrevScaledInput=DiscIntNeverNeededParam
  Add Noise : RandomNumber  Variance=1e-9  SampleTime=baseRate
  MATLAB Function : MATLAB Function  TreatAsAtomicUnit=on
  Sum : Sum  Inputs=++|
  Velocity to Position : DiscreteIntegrator  IntegratorMethod=Integration: Backward Euler  InitialCondition=drop_states_BLUE  SampleTime=-1  ICPrevOutput=DiscIntNeverNeededParam  ICPrevScaledInput=DiscIntNeverNeededParam
  states : Outport  VectorParamsAs1DForOutWhenUnconnected=off
  wires:
  control_inputs/1 -> MATLAB Function/1(control_inputs)
  Acceleration to Velocity/1 -> Velocity to Position/1
  Velocity to Position/1 -> states/1
  Add Noise/1 -> Sum/1
  MATLAB Function/1(x_ddot) -> Sum/2
  Sum/1 -> Acceleration to Velocity/1

== system MPC/Simulate Plant Dynamics/BLUE Dynamics/Calculated & Store Measured States ==
  y : Inport
  dt : Inport  Port=2
  Data Store Write1 : DataStoreWrite  DataStoreName=BLUE_Measured_States_RAW  IndexOptions=Index vector (dialog)  Indices=1  OutputSizes=1
  Data Store Write8 : DataStoreWrite  Commented=on  DataStoreName=BLUE_Measured_States  IndexOptions=Index vector (dialog)  Indices=1  OutputSizes=1
  Demux : Demux  Outputs=3
  Mux1 : Mux  Inputs=3
  Mux2 : Mux  Inputs=3
  Reshape : Reshape  OutputDimensionality=Column vector (2-D)
  Subsystem1 : Subsystem
  Subsystem2 : Subsystem
  Wrap : Subsystem
  wires:
  Demux/1 -> Mux1/1
  Wrap/1(Wrapped Angle) -> Mux1/3
  Demux/3 -> Wrap/1(Unwrapped Angle)
  Demux/2 -> Mux1/2
  Mux2/1 -> Data Store Write8/1, Data Store Write1/1
  Reshape/1 -> Subsystem1/2(y)
  Subsystem2/1(dy/dt) -> Mux2/2, Reshape/1
  y/1 -> Subsystem2/2(y), Demux/1
  dt/1 -> Subsystem1/1(dt), Subsystem2/1(dt)
  Subsystem1/1(dy/dt) -> Mux2/3
  Mux1/1 -> Mux2/1
